simulink model "UDE_Test"  (R2019b)
settings: Solver=ode4  StartTime=0.0  StopTime=tstop  FixedStep=tstep  RelTol=1e-3
values from neighbouring files (symbols this model uses):
  b_n = 5    [data.m]
  x_hat_ic = [5; -10]    [data.m]
  xic = [-5; -10]    [data.m]
settings Model: Creator=WIN10  LastModifiedBy=WIN10
settings DataIOCC: SaveOutput=off  SignalLogging=off  DSMLogging=off  SaveTime=off  ReturnWorkspaceOutputs=off

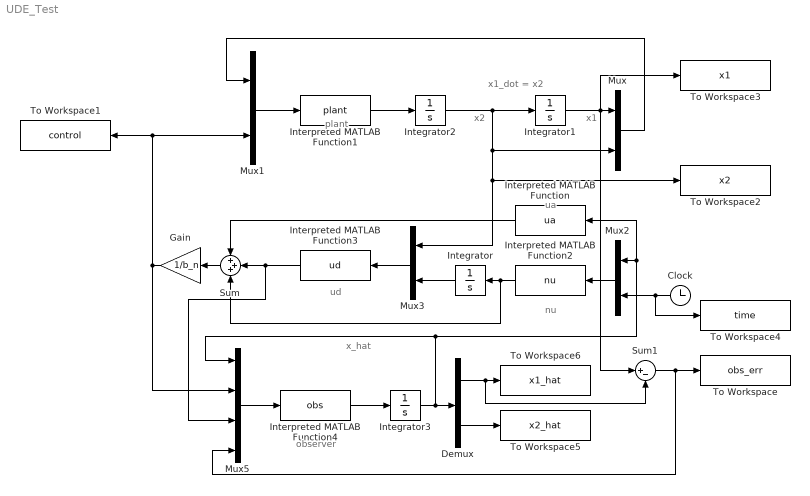
== system UDE_Test ==
  note: x_hat
  note: x1_dot = x2
  note: plant
  note: ud
  note: nu
  note: ua
  note: x1
  note: x2
  note: observer
  Clock : Clock
  Demux : Demux  Outputs=2
  Gain : Gain  Gain=1/b_n
  Integrator : Integrator
  Integrator1 : Integrator  InitialCondition=xic(1)
  Integrator2 : Integrator  InitialCondition=xic(2)
  Integrator3 : Integrator  InitialCondition=x_hat_ic
  Interpreted MATLAB Function : MATLABFcn  MATLABFcn=ua  OutputDimensions=1
  Interpreted MATLAB Function1 : MATLABFcn  MATLABFcn=plant  OutputDimensions=1
  Interpreted MATLAB Function2 : MATLABFcn  MATLABFcn=nu  OutputDimensions=1
  Interpreted MATLAB Function3 : MATLABFcn  MATLABFcn=ud  OutputDimensions=1
  Interpreted MATLAB Function4 : MATLABFcn  MATLABFcn=obs  OutputDimensions=2  Output1D=off
  Mux{,1..3} (4 alike) : Mux  Inputs=2
  Mux5 : Mux
  Sum : Sum  Inputs=+++
  Sum1 : Sum  Inputs=|+-
  To Workspace : ToWorkspace  VariableName=obs_err  SampleTime=-1
  To Workspace1 : ToWorkspace  VariableName=control  SampleTime=-1
  To Workspace2 : ToWorkspace  VariableName=x2  SampleTime=-1
  To Workspace3 : ToWorkspace  VariableName=x1  SampleTime=-1
  To Workspace4 : ToWorkspace  VariableName=time  SampleTime=-1
  To Workspace5 : ToWorkspace  VariableName=x2_hat  SampleTime=-1
  To Workspace6 : ToWorkspace  VariableName=x1_hat  SampleTime=-1
  wires:
  Interpreted MATLAB Function1/1 -> Integrator2/1
  Integrator2/1 -> Integrator1/1, To Workspace2/1, Mux3/1, Mux/2
  Integrator1/1 -> Sum1/1, To Workspace3/1, Mux/1
  Mux1/1 -> Interpreted MATLAB Function1/1
  Mux/1 -> Mux1/1
  Mux2/1 -> Interpreted MATLAB Function2/1
  Clock/1 -> To Workspace4/1, Mux2/2
  Interpreted MATLAB Function2/1 -> Sum/3, Integrator/1
  Integrator/1 -> Mux3/2
  Mux3/1 -> Interpreted MATLAB Function3/1
  Interpreted MATLAB Function/1 -> Sum/1
  Sum/1 -> Gain/1
  Interpreted MATLAB Function3/1 -> Mux5/3, Sum/2
  Gain/1 -> Mux5/2, To Workspace1/1, Mux1/2
  Mux5/1 -> Interpreted MATLAB Function4/1
  Demux/1 -> Sum1/2, To Workspace6/1
  Demux/2 -> To Workspace5/1
  Sum1/1 -> To Workspace/1, Mux5/4
  Interpreted MATLAB Function4/1 -> Integrator3/1
  Integrator3/1 -> Demux/1, Interpreted MATLAB Function/1, Mux2/1, Mux5/1
